simulink model "model"  (R2022b)
settings: Solver=FixedStepDiscrete  StartTime=0.0  StopTime=10.0  RelTol=1e-3  EnableMultiTasking=on
undefined symbols (not defined in the file or in its folder): D1, P
settings Model: DataDictionary=InterFaceDict.sldd  Creator=l33t  LastModifiedBy=l33t
settings SolverCC: AlgebraicLoopSolver=TrustRegion  AutoInsertRateTranBlk=on  InsertRTBMode=Never (minimum delay)  MaxZcPerStep=1
settings OptimizationCC: DefaultParameterBehavior=Inlined  EnhancedBackFolding=on  PassReuseOutputArgsAs=Individual arguments  ZeroExternalMemoryAtStartup=off  ZeroInternalMemoryAtStartup=off  OptimizeBlockOrder=speed  DifferentSizesBufferReuse=on  OptimizationCustomize=off  EfficientTunableParamExpr=on
settings DebuggingCC: MultiTaskDSMMsg=none  MultiTaskRateTransMsg=warning  ParameterTunabilityLossMsg=error  UnconnectedLineMsg=warning  SFMachineParentedDataDiag=warning
settings ModelReferenceCC: EnableRefExpFcnMdlSchedulingChecks=on
settings SFSimCC: MATLABDynamicMemAlloc=off
settings RTWCC: Description=AUTOSAR  SystemTargetFile=autosar.tlc  GenCodeOnly=on  TemplateMakefile=ert_default_tmf  IncludeHyperlinkInReport=on  DLArmComputeVersion=19.05
settings CodeAppCC: ForceParamTrailComments=on  IgnoreCustomStorageClasses=off  OperatorAnnotations=on  SimulinkDataObjDesc=on  SFDataObjDesc=on  InsertBlockDesc=on
settings STFCustomTargetCC: TargetLangStandard=C99 (ISO)  MultiwordLength=256  ParMdlRefBuildCompliant=on  CompOptLevelCompliant=on  IncludeMdlTerminateFcn=off  CombineOutputUpdateFcns=on  SuppressErrorStatus=on  ERTCustomFileBanners=on  SupportNonFinite=off  SupportComplex=off  SupportContinuousTime=off  SupportNonInlinedSFcns=off  RemoveResetFunc=on  MATLABClassNameForMDSCustomization=Simulink.SoftwareTarget.ERTCustomization  AutosarCompliant=on  UseToolchainInfoCompliant=on  LookupTableObjectStructAxisOrder=2,1,3,4,...  LUTObjectStructOrderEvenSpacing=Size,Table,Breakpoints  SystemTargetFile=autosar.tlc
settings ERTTargetCC: TargetLangStandard=C99 (ISO)  ConcurrentExecutionCompliant=off  IncludeMdlTerminateFcn=off  SuppressErrorStatus=on  SupportNonFinite=off  SupportComplex=off  ModelStepFunctionPrototypeControlCompliant=off  CPPClassGenCompliant=off  AutosarCompliant=on  LookupTableObjectStructAxisOrder=2,1,3,4,...  LUTObjectStructOrderEvenSpacing=Size,Table,Breakpoints  InlinedParameterPlacement=NonHierarchical  ERTCustomFileTemplate=example_file_process.tlc

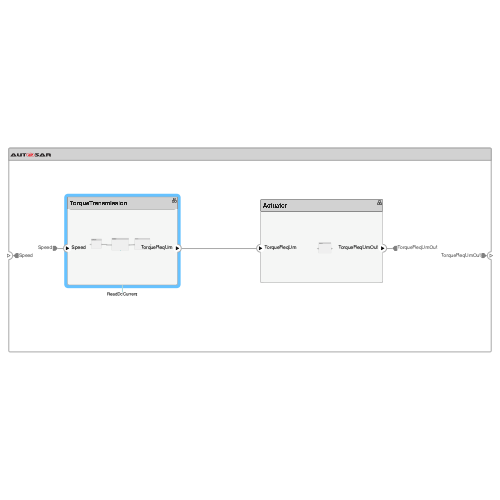
[thumbnail: Simulink's stored preview of the top-level diagram]
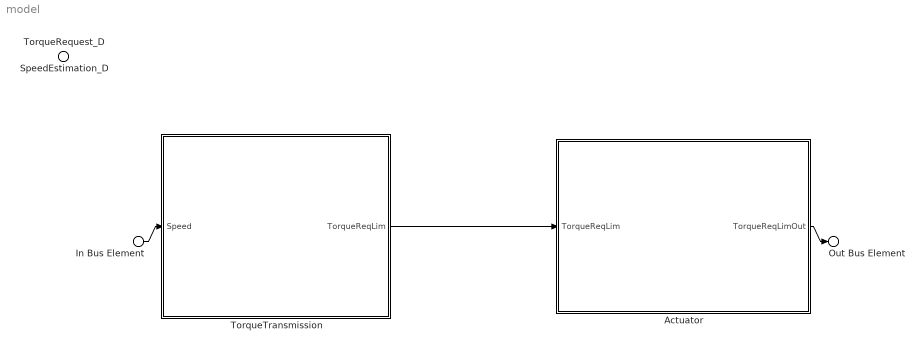
== system model ==
  In Bus Element : Inport  PortName=Speed
  SpeedEstimation_D : Inport  Port=2  OutputFunctionCall=on
  TorqueRequest_D : Inport  Port=3  OutputFunctionCall=on
  Actuator : Subsystem
      settings: PortSchema="{\"entries\":[{\"content\":{\"headerSize\":26,\"margin\":15,\"minimumSpacing\":25,\"sides\":[{\"content\":{\"connectorIds\":[\"In1\"]},\"type\":\"ConnectorPlacement.EquallySpacedRectSide\",\"uuid\":\"00703325-e225-4acb-8d9f-b9b75991ec3e\"},{\"content\":{\"connectorIds\":[\"Out1\"],\"side\":\"RIGHT\"},\"type\":\"ConnectorPlacement.EquallySpacedRectSide\",\"uuid\":\"e2ea9d97-b318-470e-bea8-ba28ee601e34\"},{\"content\":{\"connectorIds\":[],\"side\":\"TOP\"},\"type\":\"ConnectorPlacement.EquallySpacedRectSide\",\"uuid\":\"1d1f7317-a5dd-48ed-9a9f-897d6a0a8928\"}]},\"type\":\"ConnectorPlacement.EquallySpacedConnector\",\"uuid\":\"98537475-d63b-4acd-a22a-c60d95e97736\"}],\"packageUris\":[\"http://schema.mathworks.com/mf0/Connector/R2020b\"],\"version\":\"1.0\"}"
  TorqueTransmission : Subsystem
      settings: PortSchema="{\"entries\":[{\"content\":{\"headerSize\":26,\"margin\":15,\"minimumSpacing\":25,\"sides\":[{\"content\":{\"connectorIds\":[\"In1\"]},\"type\":\"ConnectorPlacement.EquallySpacedRectSide\",\"uuid\":\"00703325-e225-4acb-8d9f-b9b75991ec3e\"},{\"content\":{\"connectorIds\":[\"Out1\"],\"side\":\"RIGHT\"},\"type\":\"ConnectorPlacement.EquallySpacedRectSide\",\"uuid\":\"e2ea9d97-b318-470e-bea8-ba28ee601e34\"},{\"content\":{\"connectorIds\":[],\"side\":\"TOP\"},\"type\":\"ConnectorPlacement.EquallySpacedRectSide\",\"uuid\":\"1d1f7317-a5dd-48ed-9a9f-897d6a0a8928\"}]},\"type\":\"ConnectorPlacement.EquallySpacedConnector\",\"uuid\":\"98537475-d63b-4acd-a22a-c60d95e97736\"}],\"packageUris\":[\"http://schema.mathworks.com/mf0/Connector/R2020b\"],\"version\":\"1.0\"}"
  Out Bus Element : Outport  PortName=TorqueReqLimOut
  wires:
  TorqueTransmission/1(TorqueReqLim) -> Actuator/1(TorqueReqLim)
  In Bus Element/1 -> TorqueTransmission/1(Speed)
  Actuator/1(TorqueReqLimOut) -> Out Bus Element/1

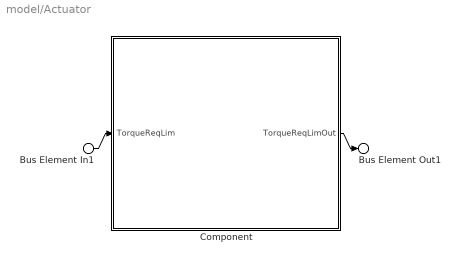
== system model/Actuator ==
  Bus Element In1 : Inport  PortName=TorqueReqLim
  Component : Subsystem
      settings: OpenFcn=disp('');  PortSchema="{\"entries\":[{\"content\":{\"headerSize\":26,\"margin\":15,\"minimumSpacing\":25,\"sides\":[{\"content\":{\"connectorIds\":[\"In1\"]},\"type\":\"ConnectorPlacement.EquallySpacedRectSide\",\"uuid\":\"00703325-e225-4acb-8d9f-b9b75991ec3e\"},{\"content\":{\"connectorIds\":[\"Out1\"],\"side\":\"RIGHT\"},\"type\":\"ConnectorPlacement.EquallySpacedRectSide\",\"uuid\":\"e2ea9d97-b318-470e-bea8-ba28ee601e34\"},{\"content\":{\"connectorIds\":[],\"side\":\"TOP\"},\"type\":\"ConnectorPlacement.EquallySpacedRectSide\",\"uuid\":\"1d1f7317-a5dd-48ed-9a9f-897d6a0a8928\"}]},\"type\":\"ConnectorPlacement.EquallySpacedConnector\",\"uuid\":\"98537475-d63b-4acd-a22a-c60d95e97736\"}],\"packageUris\":[\"http://schema.mathworks.com/mf0/Connector/R2020b\"],\"version\":\"1.0\"}"
  Bus Element Out1 : Outport  PortName=TorqueReqLimOut
  wires:
  Bus Element In1/1 -> Component/1(TorqueReqLim)
  Component/1(TorqueReqLimOut) -> Bus Element Out1/1

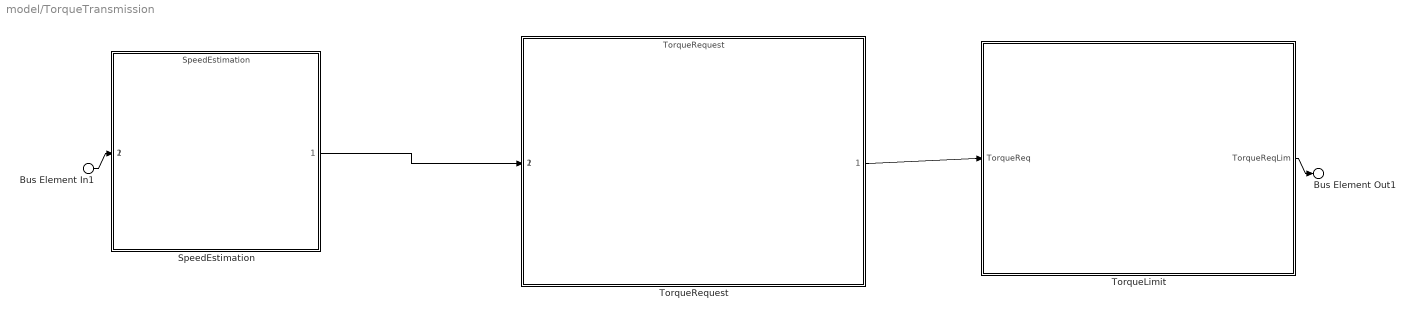
== system model/TorqueTransmission ==
  Bus Element In1 : Inport  PortName=Speed
  SpeedEstimation : ModelReference  ModelNameDialog=SpeedEstimation  SimulationMode=Normal  ScheduleRates=on  CachedPortDiscreteRates=[-1]  ModelEventPortInfo=P:D1[-1][0][0]  CodeInterface=Top model  ModelReferenceVersion=1.4
      settings: PortSchema="{\"entries\":[{\"content\":{\"headerSize\":38,\"margin\":15,\"minimumSpacing\":25,\"sides\":[{\"content\":{\"connectorIds\":[\"In1\"]},\"type\":\"ConnectorPlacement.EquallySpacedRectSide\",\"uuid\":\"00703325-e225-4acb-8d9f-b9b75991ec3e\"},{\"content\":{\"connectorIds\":[\"Out1\"],\"side\":\"RIGHT\"},\"type\":\"ConnectorPlacement.EquallySpacedRectSide\",\"uuid\":\"e2ea9d97-b318-470e-bea8-ba28ee601e34\"},{\"content\":{\"connectorIds\":[],\"side\":\"TOP\"},\"type\":\"ConnectorPlacement.EquallySpacedRectSide\",\"uuid\":\"1d1f7317-a5dd-48ed-9a9f-897d6a0a8928\"},{\"content\":{\"connectorIds\":[\"In2\"],\"side\":\"HIDDEN\"},\"type\":\"ConnectorPlacement.EquallySpacedRectSide\",\"uuid\":\"13baccb5-2292-4f78-871d-bab351dc78d5\"}]},\"type\":\"ConnectorPlacement.EquallySpacedConnector\",\"uuid\":\"98537475-d63b-4acd-a22a-c60d95e97736\"}],\"packageUris\":[\"http://schema.mathworks.com/mf0/Connector/R2020b\"],\"version\":\"1.0\"}"
  TorqueLimit : Subsystem
      settings: OpenFcn=disp('');  PortSchema="{\"entries\":[{\"content\":{\"headerSize\":26,\"margin\":15,\"minimumSpacing\":25,\"sides\":[{\"content\":{\"connectorIds\":[\"In1\"]},\"type\":\"ConnectorPlacement.EquallySpacedRectSide\",\"uuid\":\"00703325-e225-4acb-8d9f-b9b75991ec3e\"},{\"content\":{\"connectorIds\":[\"Out1\"],\"side\":\"RIGHT\"},\"type\":\"ConnectorPlacement.EquallySpacedRectSide\",\"uuid\":\"e2ea9d97-b318-470e-bea8-ba28ee601e34\"},{\"content\":{\"connectorIds\":[],\"side\":\"TOP\"},\"type\":\"ConnectorPlacement.EquallySpacedRectSide\",\"uuid\":\"1d1f7317-a5dd-48ed-9a9f-897d6a0a8928\"}]},\"type\":\"ConnectorPlacement.EquallySpacedConnector\",\"uuid\":\"98537475-d63b-4acd-a22a-c60d95e97736\"}],\"packageUris\":[\"http://schema.mathworks.com/mf0/Connector/R2020b\"],\"version\":\"1.0\"}"
  TorqueRequest : ModelReference  ModelNameDialog=TorqueRequest  SimulationMode=Normal  ScheduleRates=on  CachedPortDiscreteRates=[-1]  ModelEventPortInfo=P:D1[-1][0][0]  CodeInterface=Top model  ModelReferenceVersion=1.6
      settings: PortSchema="{\"entries\":[{\"content\":{\"headerSize\":38,\"margin\":15,\"minimumSpacing\":25,\"sides\":[{\"content\":{\"connectorIds\":[\"In1\"]},\"type\":\"ConnectorPlacement.EquallySpacedRectSide\",\"uuid\":\"00703325-e225-4acb-8d9f-b9b75991ec3e\"},{\"content\":{\"connectorIds\":[\"Out1\"],\"side\":\"RIGHT\"},\"type\":\"ConnectorPlacement.EquallySpacedRectSide\",\"uuid\":\"e2ea9d97-b318-470e-bea8-ba28ee601e34\"},{\"content\":{\"connectorIds\":[],\"side\":\"TOP\"},\"type\":\"ConnectorPlacement.EquallySpacedRectSide\",\"uuid\":\"1d1f7317-a5dd-48ed-9a9f-897d6a0a8928\"},{\"content\":{\"connectorIds\":[\"In2\"],\"side\":\"HIDDEN\"},\"type\":\"ConnectorPlacement.EquallySpacedRectSide\",\"uuid\":\"c457a32d-3575-4bef-9ee0-686ddcd58edc\"}]},\"type\":\"ConnectorPlacement.EquallySpacedConnector\",\"uuid\":\"98537475-d63b-4acd-a22a-c60d95e97736\"}],\"packageUris\":[\"http://schema.mathworks.com/mf0/Connector/R2020b\"],\"version\":\"1.0\"}"
  Bus Element Out1 : Outport  PortName=TorqueReqLim
  wires:
  TorqueLimit/1(TorqueReqLim) -> Bus Element Out1/1
  Bus Element In1/1 -> SpeedEstimation/1
  SpeedEstimation/1 -> TorqueRequest/1
  TorqueRequest/1 -> TorqueLimit/1(TorqueReq)

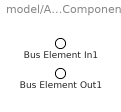
== system model/Actuator/Component ==
  Bus Element In1 : Inport  PortName=TorqueReqLim
  Bus Element Out1 : Outport  PortName=TorqueReqLimOut

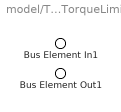
== system model/TorqueTransmission/TorqueLimit ==
  Bus Element In1 : Inport  PortName=TorqueReq
  Bus Element Out1 : Outport  PortName=TorqueReqLim
